simulink model "flexible_spacecraft"  (R2015b)
settings: Solver=VariableStepAuto  StartTime=0.0  StopTime=2000  FixedStep=0.1  MaxStep=0.01  RelTol=1e-3
undefined symbols (not defined in the file): delta, J, k1, k2, lambda
libraries: simulink x1, vrlib x1
settings Model: SimulationMode=accelerator  Creator=DNikolaev  LastModifiedBy=DNikolaev

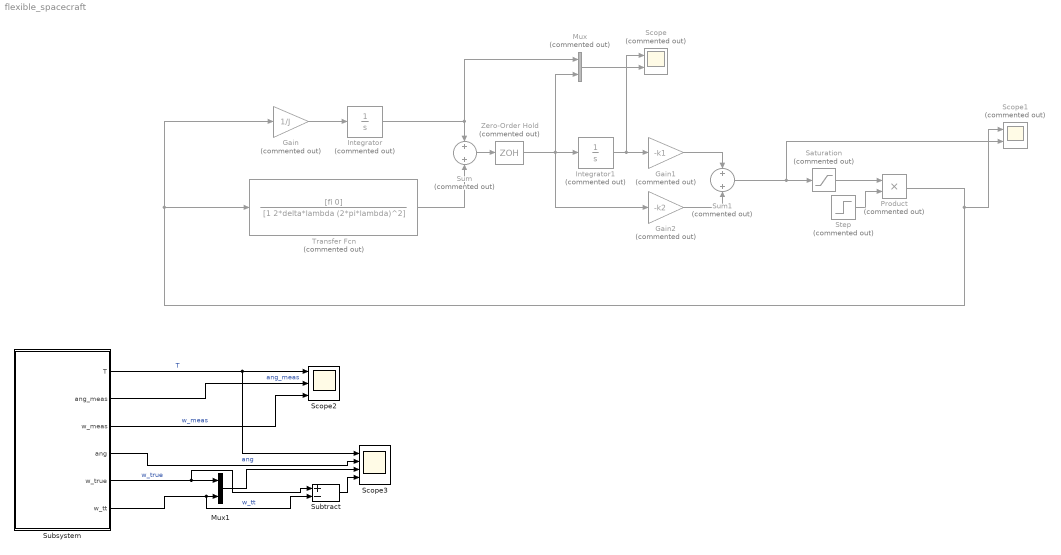
== system flexible_spacecraft ==
  Gain : Gain  Commented=on  Gain=1/J
  Gain1 : Gain  Commented=on  Gain=-k1
  Gain2 : Gain  Commented=on  Gain=-k2
  Integrator : Integrator  Commented=on
  Integrator1 : Integrator  Commented=on  InitialCondition=0.000001
  Mux : Mux  Commented=on  Inputs=2
  Mux1 : Mux  Inputs=2
  Product : Product  Commented=on
  Saturation : Saturate  Commented=on  UpperLimit=0.1  LowerLimit=-0.1
  Scope : Scope  Commented=on  NumInputPorts=2
  Scope1 : Scope  Commented=on  NumInputPorts=2
  Scope2 : Scope  NumInputPorts=3
  Scope3 : Scope  NumInputPorts=4
  Step : Step  Commented=on  Time=10  SampleTime=0
  Subsystem : Subsystem  mask{fi=[0 0.1 0], J=diag([1900 1900 150]), delta=0.2, lambda=0.5, init_ang=[0 deg2rad(-177) 0], init_vel=[0 0 0], k1=3e-3*1900, k2=0.3*1900}
      mask prompts: fi "fi-vect"; J "Inertia"; lambda "lambda, Hz"; init_ang "Initial angle"; init_vel "Initial velocity"
  Subtract : Sum  Inputs=+-
  Sum : Sum  Commented=on  Inputs=+|+
  Sum1 : Sum  Commented=on
  Transfer Fcn : TransferFcn  Commented=on  Numerator=[fi 0]  Denominator=[1 2*delta*lambda (2*pi*lambda)^2]
  Zero-Order Hold : ZeroOrderHold  Commented=on  SampleTime=0.1
  wires:
  Integrator/1 -> Mux/1, Sum/1
  Transfer Fcn/1 -> Sum/2
  Gain/1 -> Integrator/1
  Sum/1 -> Zero-Order Hold/1
  Integrator1/1 -> Scope/1, Gain1/1
  Gain1/1 -> Sum1/1
  Gain2/1 -> Sum1/2
  Saturation/1 -> Product/1
  Step/1 -> Product/2
  Product/1 -> Gain/1, Transfer Fcn/1, Scope1/1
  Sum1/1 -> Scope1/2, Saturation/1
  Mux/1 -> Scope/2
  Zero-Order Hold/1 -> Mux/2, Gain2/1, Integrator1/1
  Subsystem/2(ang_meas) -> Scope2/2  "ang_meas"
  Subsystem/1(T) -> Scope3/1, Scope2/1  "T"
  Subsystem/3(w_meas) -> Scope2/3  "w_meas"
  Subsystem/4(ang) -> Scope3/2  "ang"
  Subsystem/5(w_true) -> Subtract/1, Mux1/1  "w_true"
  Subsystem/6(w_tt) -> Subtract/2, Mux1/2  "w_tt"
  Mux1/1 -> Scope3/3
  Subtract/1 -> Scope3/4

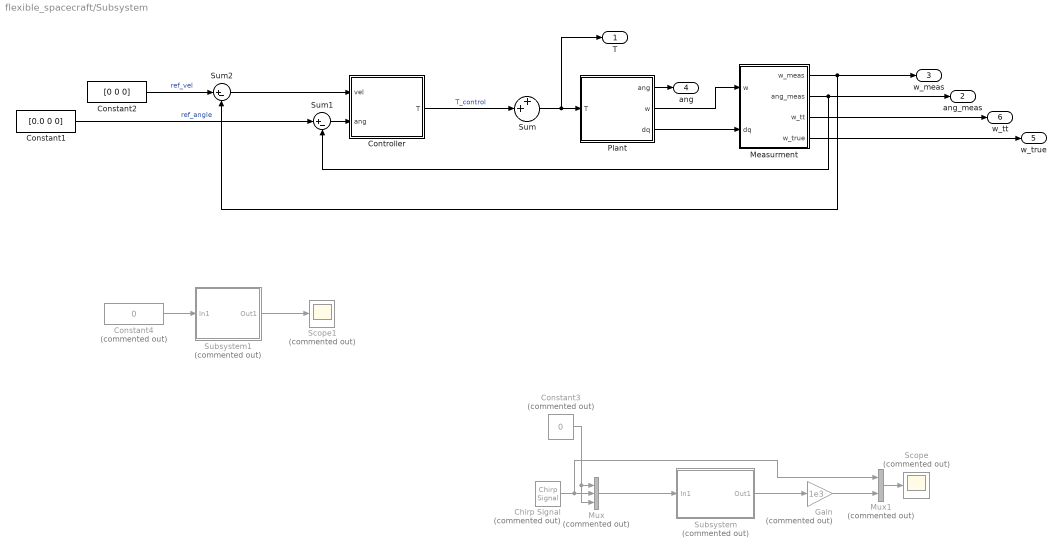
== system flexible_spacecraft/Subsystem ==
  Chirp Signal : simulink/Sources/Chirp Signal  Commented=on  f1=0  T=100  f2=10
  Constant1 : Constant  Value=[0.0 0 0]
  Constant2 : Constant  Value=[0 0 0]
  Constant3 : Constant  Commented=on  Value=0
  Constant4 : Constant  Commented=on  Value=0  SampleTime=0.1
  Controller : Subsystem
  Gain : Gain  Commented=on  Gain=1e3
  Measurment : Subsystem
  Mux : Mux  Commented=on  Inputs=3
  Mux1 : Mux  Commented=on  Inputs=2
  Plant : Subsystem
  Scope : Scope  Commented=on
  Scope1 : Scope  Commented=on
  Subsystem : Subsystem  Commented=on
  Subsystem1 : Subsystem  Commented=on
  Sum : Sum  Inputs=++|
  Sum1 : Sum  Inputs=|+-
  Sum2 : Sum  Inputs=|+-
  T : Outport
  ang_meas : Outport  Port=2
  w_meas : Outport  Port=3
  ang : Outport  Port=4
  w_true : Outport  Port=5
  w_tt : Outport  Port=6
  wires:
  Sum/1 -> T/1, Plant/1(T)
  Plant/2(w) -> Measurment/1(w)
  Plant/3(dq) -> Measurment/2(dq)
  Measurment/1(w_meas) -> Sum2/2, w_meas/1
  Measurment/2(ang_meas) -> Sum1/2, ang_meas/1
  Controller/1(T) -> Sum/2  "T_control"
  Plant/1(ang) -> ang/1
  Sum2/1 -> Controller/1(vel)
  Sum1/1 -> Controller/2(ang)
  Constant1/1 -> Sum1/1  "ref_angle"
  Constant2/1 -> Sum2/1  "ref_vel"
  Measurment/4(w_true) -> w_true/1
  Measurment/3(w_tt) -> w_tt/1
  Chirp Signal/1 -> Mux1/1, Mux/2
  Mux/1 -> Subsystem/1(In1)
  Subsystem/1(Out1) -> Gain/1
  Constant3/1 -> Mux/3, Mux/1
  Mux1/1 -> Scope/1
  Gain/1 -> Mux1/2
  Subsystem1/1(Out1) -> Scope1/1
  Constant4/1 -> Subsystem1/1(In1)

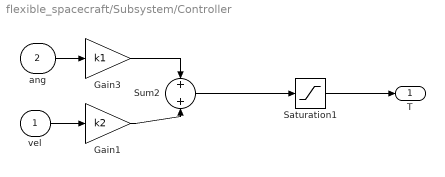
== system flexible_spacecraft/Subsystem/Controller ==
  vel : Inport
  ang : Inport  Port=2
  Gain1 : Gain  Gain=k2
  Gain3 : Gain  Gain=k1
  Saturation1 : Saturate  UpperLimit=0.1  LowerLimit=-0.1
  Sum2 : Sum
  T : Outport
  wires:
  vel/1 -> Gain1/1
  Gain3/1 -> Sum2/1
  Saturation1/1 -> T/1
  ang/1 -> Gain3/1
  Sum2/1 -> Saturation1/1
  Gain1/1 -> Sum2/2

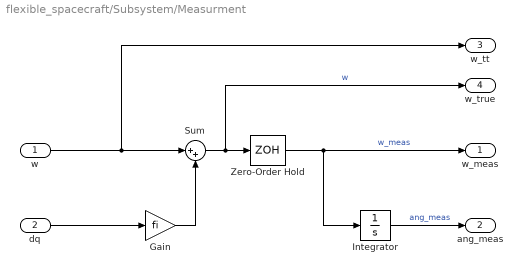
== system flexible_spacecraft/Subsystem/Measurment ==
  w : Inport
  dq : Inport  Port=2
  Gain : Gain  Gain=fi
  Integrator : Integrator  InitialCondition=init_ang
  Sum : Sum  Inputs=|++
  Zero-Order Hold : ZeroOrderHold  SampleTime=0.1
  w_meas : Outport
  ang_meas : Outport  Port=2
  w_tt : Outport  Port=3
  w_true : Outport  Port=4
  wires:
  w/1 -> Sum/1, w_tt/1
  dq/1 -> Gain/1
  Gain/1 -> Sum/2
  Sum/1 -> w_true/1, Zero-Order Hold/1  "w"
  Integrator/1 -> ang_meas/1  "ang_meas"
  Zero-Order Hold/1 -> w_meas/1, Integrator/1  "w_meas"

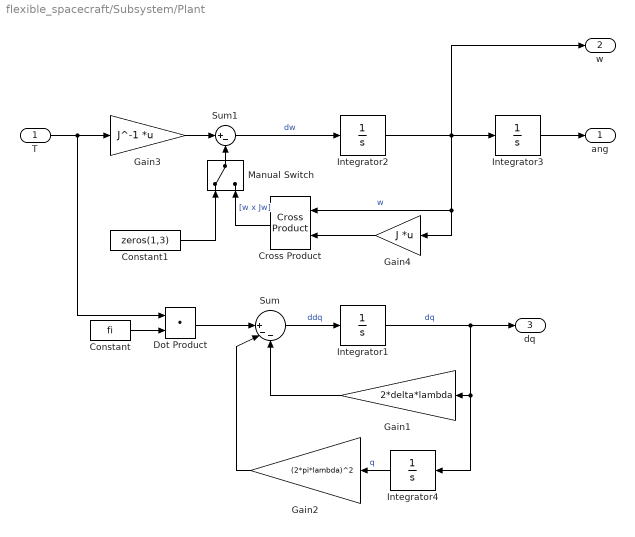
== system flexible_spacecraft/Subsystem/Plant ==
  T : Inport
  Constant : Constant  Value=fi
  Constant1 : Constant  Value=zeros(1,3)
  Cross Product : vrlib/Utilities/Cross Product
  Dot Product : DotProduct  InputSameDT=on  OutDataTypeStr=Inherit: Inherit via internal rule
  Gain1 : Gain  Gain=2*delta*lambda
  Gain2 : Gain  Gain=(2*pi*lambda)^2
  Gain3 : Gain  Gain=J^-1  Multiplication=Matrix(K*u)
  Gain4 : Gain  Gain=J  Multiplication=Matrix(K*u)
  Integrator1 : Integrator
  Integrator2 : Integrator  InitialCondition=init_vel
  Integrator3 : Integrator  InitialCondition=init_ang
  Integrator4 : Integrator
  Manual Switch : ManualSwitch
  Sum : Sum  Inputs=||+--
  Sum1 : Sum  Inputs=|+-
  ang : Outport
  w : Outport  Port=2
  dq : Outport  Port=3
  wires:
  T/1 -> Dot Product/1, Gain3/1
  Gain3/1 -> Sum1/1
  Integrator2/1 -> Integrator3/1, Cross Product/1, Gain4/1, w/1  "w"
  Constant/1 -> Dot Product/2
  Integrator4/1 -> Gain2/1  "q"
  Gain2/1 -> Sum/2
  Gain1/1 -> Sum/3
  Dot Product/1 -> Sum/1
  Sum/1 -> Integrator1/1  "ddq"
  Integrator1/1 -> dq/1, Integrator4/1, Gain1/1  "dq"
  Sum1/1 -> Integrator2/1  "dw"
  Cross Product/1 -> Manual Switch/2  "[w x Jw]"
  Gain4/1 -> Cross Product/2
  Integrator3/1 -> ang/1
  Manual Switch/1 -> Sum1/2
  Constant1/1 -> Manual Switch/1

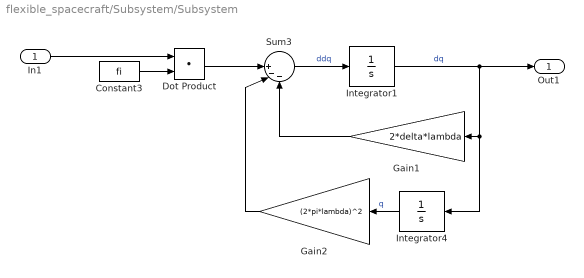
== system flexible_spacecraft/Subsystem/Subsystem ==
  In1 : Inport
  Constant3 : Constant  Value=fi
  Dot Product : DotProduct  InputSameDT=on  OutDataTypeStr=Inherit: Inherit via internal rule
  Gain1 : Gain  Gain=2*delta*lambda
  Gain2 : Gain  Gain=(2*pi*lambda)^2
  Integrator1 : Integrator
  Integrator4 : Integrator
  Sum3 : Sum  Inputs=||+--
  Out1 : Outport
  wires:
  Sum3/1 -> Integrator1/1  "ddq"
  In1/1 -> Dot Product/1
  Integrator1/1 -> Out1/1, Integrator4/1, Gain1/1  "dq"
  Gain1/1 -> Sum3/3
  Gain2/1 -> Sum3/2
  Constant3/1 -> Dot Product/2
  Dot Product/1 -> Sum3/1
  Integrator4/1 -> Gain2/1  "q"

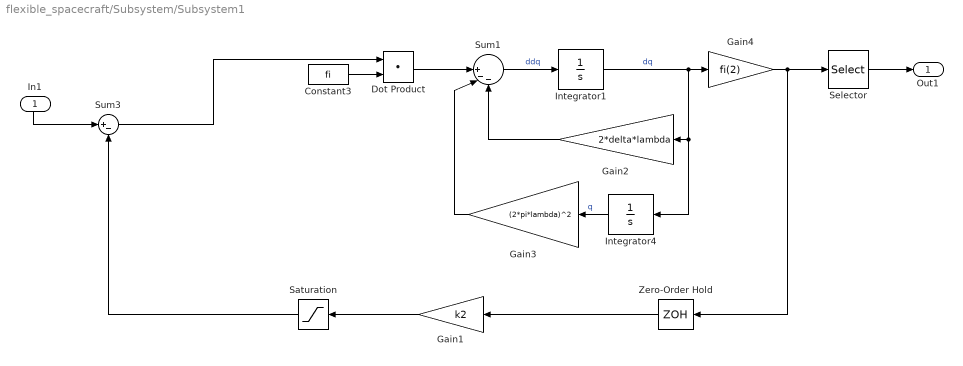
== system flexible_spacecraft/Subsystem/Subsystem1 ==
  In1 : Inport
  Constant3 : Constant  Value=fi
  Dot Product : DotProduct  InputSameDT=on  OutDataTypeStr=Inherit: Inherit via internal rule
  Gain1 : Gain  Gain=k2
  Gain2 : Gain  Gain=2*delta*lambda
  Gain3 : Gain  Gain=(2*pi*lambda)^2
  Gain4 : Gain  Gain=fi(2)
  Integrator1 : Integrator  InitialCondition=1
  Integrator4 : Integrator
  Saturation : Saturate  UpperLimit=0.1  LowerLimit=-0.1
  Selector : Selector  InputPortWidth=3  IndexOptions=Index vector (dialog)  Indices=2  OutputSizes=1
  Sum1 : Sum  Inputs=||+--
  Sum3 : Sum  Inputs=|+-
  Zero-Order Hold : ZeroOrderHold  SampleTime=0.1
  Out1 : Outport
  wires:
  Gain1/1 -> Saturation/1
  In1/1 -> Sum3/1
  Sum1/1 -> Integrator1/1  "ddq"
  Sum3/1 -> Dot Product/1
  Integrator1/1 -> Integrator4/1, Gain2/1, Gain4/1  "dq"
  Gain2/1 -> Sum1/3
  Gain3/1 -> Sum1/2
  Constant3/1 -> Dot Product/2
  Dot Product/1 -> Sum1/1
  Integrator4/1 -> Gain3/1  "q"
  Gain4/1 -> Selector/1, Zero-Order Hold/1
  Zero-Order Hold/1 -> Gain1/1
  Selector/1 -> Out1/1
  Saturation/1 -> Sum3/2
